simulink model "double_integrator_simulink"  (R2024b)
settings: Solver=VariableStepAuto  StartTime=0.0  StopTime=10.0  RelTol=1e-3
settings Model: Creator=StavrosAlx  LastModifiedBy=StavrosAlx

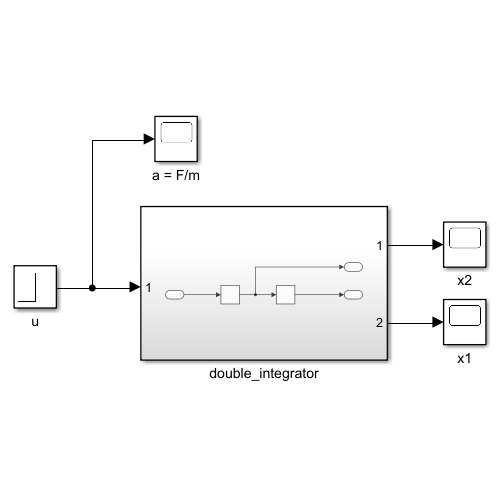
[thumbnail: Simulink's stored preview of the top-level diagram]
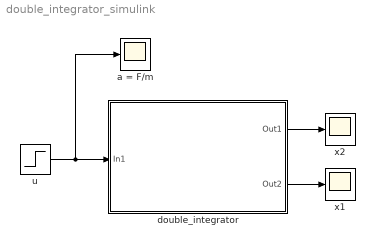
== system double_integrator_simulink ==
  a = F/m : Scope
  double_integrator : Subsystem
  u : Step  SampleTime=0
  x1 : Scope
  x2 : Scope
  wires:
  u/1 -> a = F/m/1, double_integrator/1(In1)
  double_integrator/1(Out1) -> x2/1
  double_integrator/2(Out2) -> x1/1

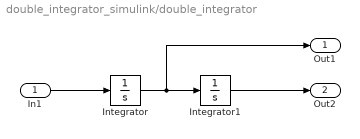
== system double_integrator_simulink/double_integrator ==
  In1 : Inport
  Integrator : Integrator
  Integrator1 : Integrator
  Out1 : Outport
  Out2 : Outport  Port=2
  wires:
  Integrator/1 -> Out1/1, Integrator1/1
  In1/1 -> Integrator/1
  Integrator1/1 -> Out2/1
